simulink model "tunning"  (R2021a)
settings: Solver=VariableStepAuto  StartTime=0.0  StopTime=1  RelTol=1e-3
values from neighbouring files (symbols this model uses):
  B = x(2)    [optimize_system.m]
  K = x(1)    [optimize_system.m]
settings Model: Creator=nathanielgoldfarb  LastModifiedBy=nathanielgoldfarb

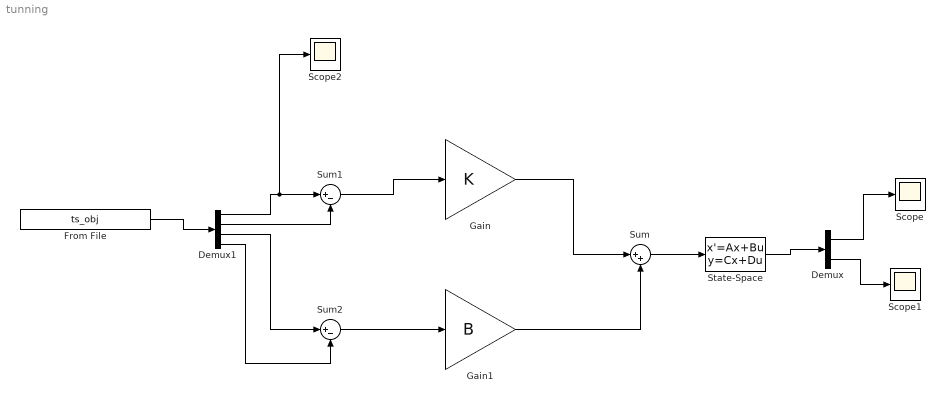
== system tunning ==
  Demux : Demux  Outputs=2
  Demux1 : Demux
  From File : FromFile  FileName=ts_obj  InterpolationWithinTimeRange=Zero order hold  ExtrapolationAfterLastDataPoint=Hold last value
  Gain : Gain  Gain=K
  Gain1 : Gain  Gain=B
  Scope : Scope
  Scope1 : Scope
  Scope2 : Scope
  State-Space : StateSpace  A=[ 0 1; 0 0]  B=[0; 1]  C=eye(2)  D=[0;0]  InitialCondition=0
  Sum : Sum  Inputs=|++
  Sum1 : Sum  Inputs=|+-
  Sum2 : Sum  Inputs=|+-
  wires:
  Gain/1 -> Sum/1
  Gain1/1 -> Sum/2
  Sum/1 -> State-Space/1
  State-Space/1 -> Demux/1
  Demux/2 -> Scope1/1
  Demux/1 -> Scope/1
  From File/1 -> Demux1/1
  Demux1/1 -> Scope2/1, Sum1/1
  Demux1/2 -> Sum1/2
  Demux1/3 -> Sum2/1
  Demux1/4 -> Sum2/2
  Sum1/1 -> Gain/1
  Sum2/1 -> Gain1/1
